simulink model "lab2test"  (R2014a)
settings: Solver=FixedStepDiscrete  StartTime=0.0  StopTime=Inf  FixedStep=sampletime  RelTol=1e-3
libraries: dspsrcs4 x1, dspindex x1, dspvision x1, dspsnks4 x1
settings Model: Creator=micro386  LastModifiedBy=micro386

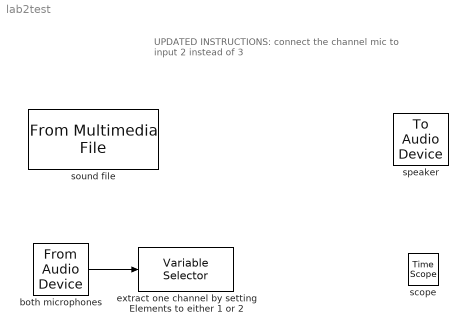
== system lab2test ==
  note: UPDATED INSTRUCTIONS:
      | connect the channel mic to input 2 instead of 3
  both microphones : dspsrcs4/From Audio Device  deviceName=FCA1616 Mic 1/2 (3- Behringer FCA1616 WDM)  numChannels=2  sampleRate=1/sampletime  deviceDatatype=Determine from output data type  autoBufferSize=on  bufferSize=4096  queueDuration=0.1  frameSize=1024  outputDatatype=double  defaultInputChannelMapping=on  inputChannelMapping=1:2
  extract one channel by setting Elements to either 1 or 2 : dspindex/Variable Selector  NumInputs=1  rowsOrCols=Columns  IdxMode=Fixed  Elements=2  ZerOneIdxMode=One-based  errmode=Clip Index  FillMode=on  FillValues=0
  "scope " : TimeScope  DefaultConfigurationName=spbscopes.TimeScopeBlockCfg
  sound file : dspvision/From Multimedia File  inputFilename=guns.wav  loop=on  numPlays=inf  outputStreams=Audio only  videoDataType=single  audioDataType=double  inheritSampleTime=on  userDefinedSampleTime=1/30  noAudioOutput=off  isIntensityVideo=off  fourcc=RGB  colorVideoFormat=Separate color signals  outputEOF=off  dataOrg=Column-major  audioFrameSize=1024  computeAudioFrameSize=off  outSamplingMode=Frame based
  "speaker " : dspsnks4/To Audio Device  deviceName=FCA1616 Line 3/4 (3- Behringer FCA1616 WDM)  inheritSampleRate=off  sampleRate=1/sampletime  deviceDatatype=Determine from input data type  autoBufferSize=on  bufferSize=4096  queueDuration=0.1  defaultOutputChannelMapping=on  outputChannelMapping=1:2
  wires:
  both microphones/1 -> extract one channel by setting Elements to either 1 or 2/1
